simulink model "Colas_bloqueo"  (R2023a)
settings: Solver=VariableStepAuto  StartTime=0.0  StopTime=30  RelTol=1e-3
undefined symbols (not defined in the file or in its folder): m, n
settings Model: Creator=santi  LastModifiedBy=santi

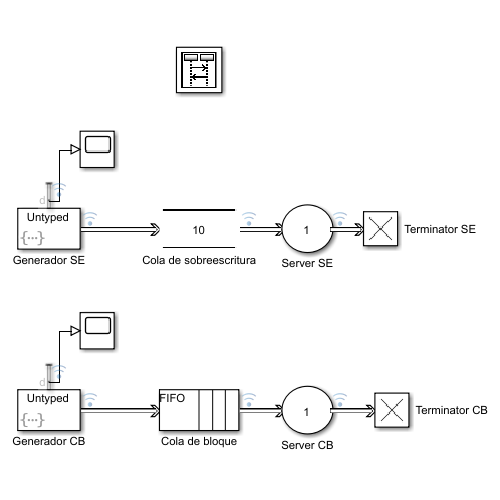
[thumbnail: Simulink's stored preview of the top-level diagram]
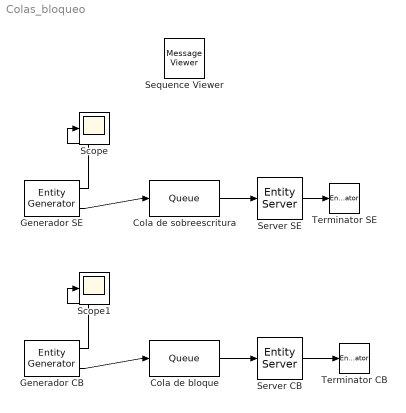
== system Colas_bloqueo ==
  Cola de bloque : Queue  InputPortMessageModes=m  OutputPortMessageModes=m  Capacity=10
  Cola de sobreescritura : Queue  InputPortMessageModes=m  OutputPortMessageModes=m  OverwriteOldest=on  Capacity=10
  Generador CB : EntityGenerator  OutputPortMessageModes=n,m  GenerateAction=entity = rand();  AttributeName=entity  NumberEntitiesDeparted=on  EntityTypeName=Entity  DataInitialValue=1
      settings: OutputPortMap=o0,o3
  Generador SE : EntityGenerator  OutputPortMessageModes=n,m  GenerateAction=entity = rand();  AttributeName=entity  NumberEntitiesDeparted=on  EntityTypeName=Entity  DataInitialValue=1
      settings: OutputPortMap=o0,o3
  Scope : Scope
  Scope1 : Scope
  Sequence Viewer : MessageViewer  History=1000  SavedRootId=#
  Server CB : EntityServer  InputPortMessageModes=m  OutputPortMessageModes=m  Capacity=1  ServiceTimeValue=25.0
  Server SE : EntityServer  InputPortMessageModes=m  OutputPortMessageModes=m  Capacity=1  ServiceTimeValue=25
  Terminator CB : EntityTerminator  InputPortMessageModes=m
  Terminator SE : EntityTerminator  InputPortMessageModes=m
  wires:
  Generador SE/2 -> Cola de sobreescritura/1
  Generador SE/1 -> Scope/1
  Cola de sobreescritura/1 -> Server SE/1
  Cola de bloque/1 -> Server CB/1
  Generador CB/1 -> Scope1/1
  Generador CB/2 -> Cola de bloque/1
  Server CB/1 -> Terminator CB/1
  Server SE/1 -> Terminator SE/1
